simulink library "csu_pvs_pressurant_valve_switch_lib"  (R2014b)
settings: Solver=ode45  StartTime=0.0  StopTime=10.0  RelTol=1e-3
undefined symbols (not defined in the file): act_full_on_duration
libraries: simulink x2, util_info_lib x1, util_event_lib x1, util_common_lib x1
settings Model: Creator=escrane  LastModifiedBy=mstewart

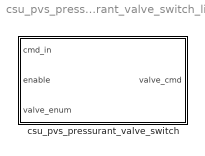
== system csu_pvs_pressurant_valve_switch_lib ==
  csu_pvs_pressurant_valve_switch : Subsystem  mask{open_duration=act_full_on_duration, closed_duration=0, event_id=22}
      mask prompts: open_duration "Commanded duration when valve OPEN"; closed_duration "Commanded duration when valve CLOSE"; event_id "Event Message ID (num > 21)"

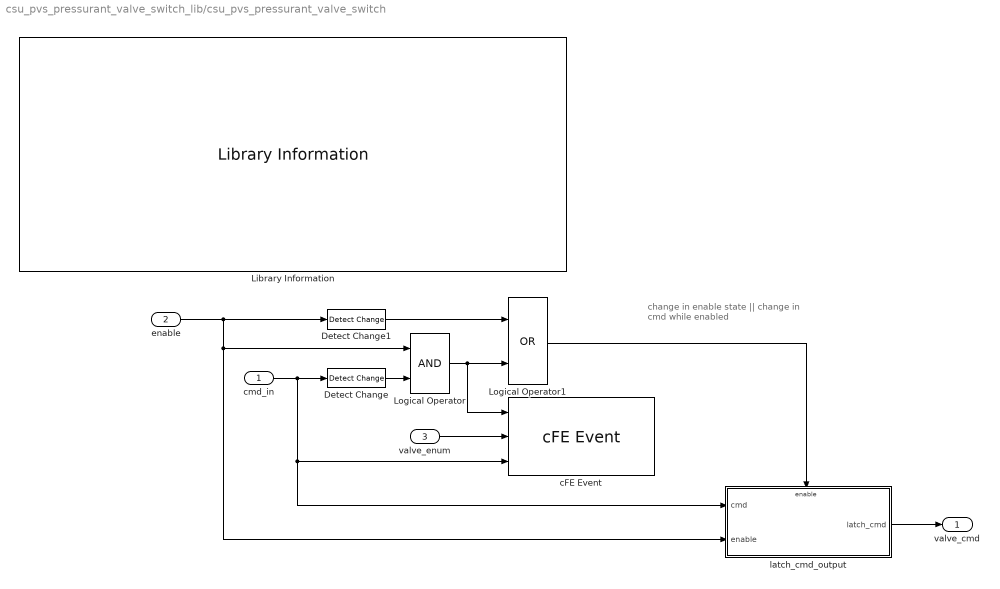
== system csu_pvs_pressurant_valve_switch_lib/csu_pvs_pressurant_valve_switch ==
  note: change in enable state
      | ||
      | change in cmd while enabled
  cmd_in : Inport
  enable : Inport  Port=2
  valve_enum : Inport  Port=3
  Detect Change : simulink/Logic and Bit Operations/Detect Change  vinit=0  InputProcessing=Inherited  OutDataTypeStr=boolean
  Detect Change1 : simulink/Logic and Bit Operations/Detect Change  vinit=0  InputProcessing=Inherited  OutDataTypeStr=boolean
  Library Information : util_info_lib/Library Information  owner='NONE'
  Logical Operator : Logic  AllPortsSameDT=off  OutDataTypeStr=boolean
  Logical Operator1 : Logic  Operator=OR  AllPortsSameDT=off  OutDataTypeStr=boolean
  cFE Event : util_event_lib/cFE Event  event_message='Changing state of %s valve to %s'  event_id=event_id  event_severity=INFORMATION  event_use_enums=on  event_enum_types={'enum_mtv_press_valve_names','enum_valve_state'}
  latch_cmd_output : Subsystem
  valve_cmd : Outport
  wires:
  valve_enum/1 -> cFE Event/2
  Detect Change/1 -> Logical Operator/2
  enable/1 -> latch_cmd_output/2(enable), Logical Operator/1, Detect Change1/1
  Logical Operator1/1 -> latch_cmd_output/Enable
  latch_cmd_output/1(latch_cmd) -> valve_cmd/1
  Logical Operator/1 -> Logical Operator1/2, cFE Event/1
  Detect Change1/1 -> Logical Operator1/1
  cmd_in/1 -> cFE Event/3, latch_cmd_output/1(cmd), Detect Change/1

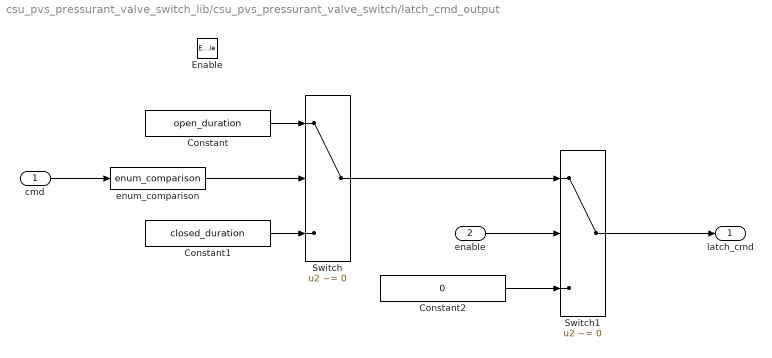
== system csu_pvs_pressurant_valve_switch_lib/csu_pvs_pressurant_valve_switch/latch_cmd_output ==
  cmd : Inport
  enable : Inport  Port=2
  Enable : EnablePort
  Constant : Constant  Value=open_duration  OutDataTypeStr=uint8
  Constant1 : Constant  Value=closed_duration  OutDataTypeStr=uint8
  Constant2 : Constant  Value=0  OutDataTypeStr=uint8
  Switch : Switch  Criteria=u2 ~= 0
  Switch1 : Switch  Criteria=u2 ~= 0
  enum_comparison : util_common_lib/enum_comparison  comparison_type===
  latch_cmd : Outport  InitialOutput=0
  wires:
  cmd/1 -> enum_comparison/1
  enum_comparison/1 -> Switch/2
  Constant/1 -> Switch/1
  Constant1/1 -> Switch/3
  enable/1 -> Switch1/2
  Switch/1 -> Switch1/1
  Constant2/1 -> Switch1/3
  Switch1/1 -> latch_cmd/1
